simulink model "untitled"  (R2017a)
settings: Solver=VariableStepAuto  StartTime=0.0  StopTime=10.0  RelTol=1e-3
settings Model: Creator=bruno  LastModifiedBy=bruno

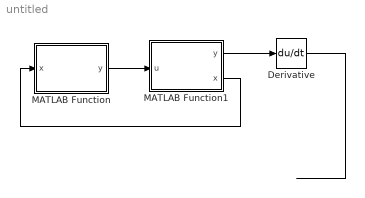
== system untitled ==
  Derivative : Derivative
  MATLAB Function : MATLAB Function  TreatAsAtomicUnit=on
  MATLAB Function1 : MATLAB Function  TreatAsAtomicUnit=on
  wires:
  MATLAB Function/1(y) -> MATLAB Function1/1(u)
  MATLAB Function1/1(y) -> Derivative/1
  MATLAB Function1/2(x) -> MATLAB Function/1(x)
  Derivative/1 -> ?

== matlab function untitled/MATLAB Function1 ==
  data: y output; x output; u input
function [y, x] = fcn(u)

== matlab function untitled/MATLAB Function ==
  data: x input; y output
function y = fcn(x)

y = u;
